simulink model "exp1_local_rendering_stg2"  (R2025a)
settings: Solver=ode4  StartTime=0.0  StopTime=0.5  FixedStep=1e-4  RelTol=1e-3
values from neighbouring files (symbols this model uses):
  Ts = T(T.classCode == 0,:)    [exp1_sweep_final.m]
undefined symbols (not defined in the file or in its folder): a, b_eq, Bc, I_eq, k_eq, Kc, r_h, r_m, r_s, vM0, xM0
settings Model: Creator=ekaitz  LastModifiedBy=ekaitz

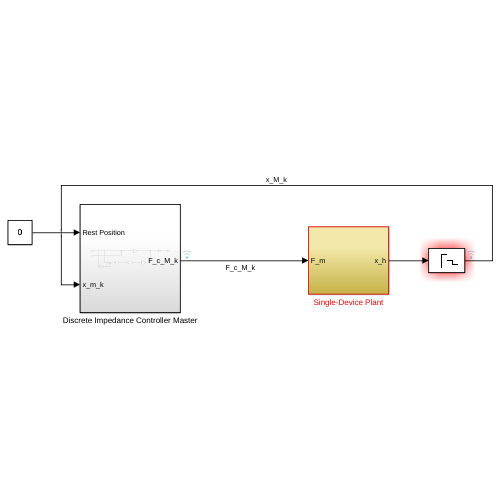
[thumbnail: Simulink's stored preview of the top-level diagram]
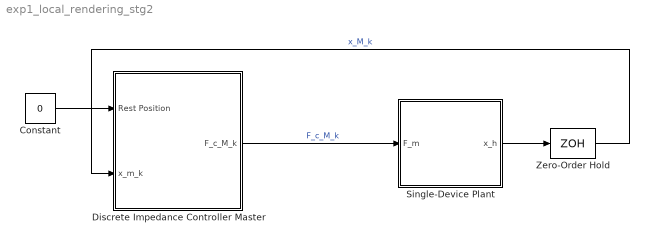
== system exp1_local_rendering_stg2 ==
  Constant : Constant  Value=0
  Discrete Impedance Controller Master : Subsystem
  Single-Device Plant : Subsystem
  Zero-Order Hold : ZeroOrderHold  SampleTime=Ts
  wires:
  Constant/1 -> Discrete Impedance Controller Master/1(Rest Position)
  Single-Device Plant/1(x_h) -> Zero-Order Hold/1
  Zero-Order Hold/1 -> Discrete Impedance Controller Master/2(x_m_k)  "x_M_k"
  Discrete Impedance Controller Master/1(F_c_M_k) -> Single-Device Plant/1(F_m)  "F_c_M_k"

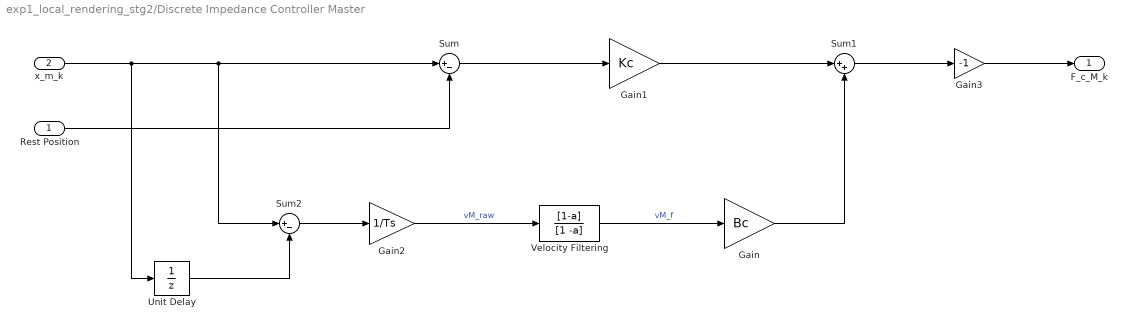
== system exp1_local_rendering_stg2/Discrete Impedance Controller Master ==
  Rest Position : Inport
  x_m_k : Inport  Port=2
  Gain : Gain  Gain=Bc
  Gain1 : Gain  Gain=Kc
  Gain2 : Gain  Gain=1/Ts
  Gain3 : Gain  Gain=-1
  Sum : Sum  Inputs=|+-
  Sum1 : Sum  Inputs=|++
  Sum2 : Sum  Inputs=|+-
  Unit Delay : UnitDelay  InitialCondition=xM0  SampleTime=Ts  HasFrameUpgradeWarning=on
  Velocity Filtering : DiscreteTransferFcn  Numerator=[1-a]  Denominator=[1 -a]
  F_c_M_k : Outport
  wires:
  Sum/1 -> Gain1/1
  Gain1/1 -> Sum1/1
  Gain/1 -> Sum1/2
  Sum1/1 -> Gain3/1
  x_m_k/1 -> Unit Delay/1, Sum2/1, Sum/1
  Unit Delay/1 -> Sum2/2
  Sum2/1 -> Gain2/1
  Rest Position/1 -> Sum/2
  Gain2/1 -> Velocity Filtering/1  "vM_raw"
  Velocity Filtering/1 -> Gain/1  "vM_f"
  Gain3/1 -> F_c_M_k/1

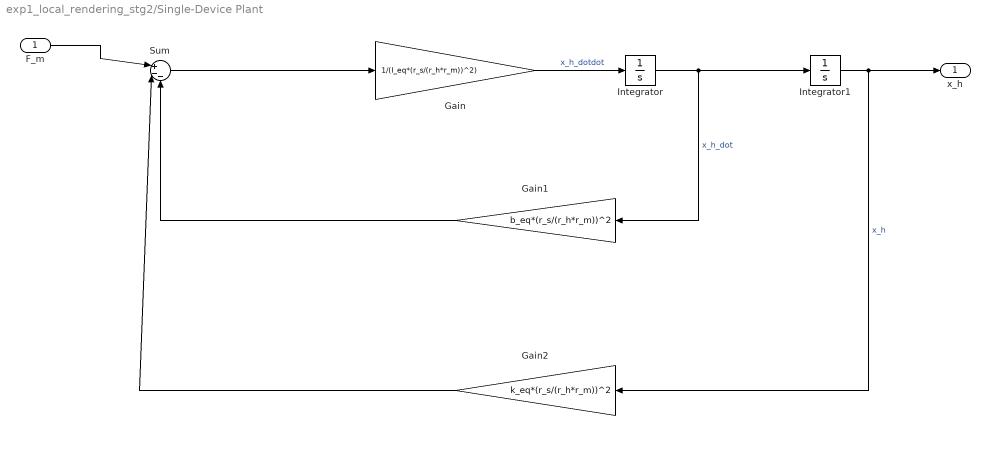
== system exp1_local_rendering_stg2/Single-Device Plant ==
  F_m : Inport
  Gain : Gain  Gain=1/(I_eq*(r_s/(r_h*r_m))^2)
  Gain1 : Gain  Gain=b_eq*(r_s/(r_h*r_m))^2
  Gain2 : Gain  Gain=k_eq*(r_s/(r_h*r_m))^2
  Integrator : Integrator  InitialCondition=vM0
  Integrator1 : Integrator  InitialCondition=xM0
  Sum : Sum  Inputs=|+--
  x_h : Outport
  wires:
  Gain2/1 -> Sum/2
  Gain/1 -> Integrator/1  "x_h_dotdot"
  F_m/1 -> Sum/1
  Integrator1/1 -> x_h/1, Gain2/1  "x_h"
  Gain1/1 -> Sum/3
  Sum/1 -> Gain/1
  Integrator/1 -> Gain1/1, Integrator1/1  "x_h_dot"
